simulink model "partialForceControlSim"  (Simulink 7.7)
settings: Solver=FixedStepDiscrete  StartTime=0.0  StopTime=inf  FixedStep=1  RelTol=1e-3
InitFcn:
  | initPartialForceControlSim;
values from neighbouring files (symbols this model uses):
  k_f = diag([k_f_linear k_f_rotatio])    [initPartialForceControl.m]
  k_pst = [ diag([k_pst_torso k_pst_arm k_pst_arm k_pst_leg k_pst_leg])    0*eye(25)   0*eye(25)]    [initPartialForceControl.m]    (also in initSharedMem.m)
  nc = 6    [initPartialForceControl.m]    (also in initSharedMem.m = 12)
  nj = 25    [initMonitor.m]    (also in initPartialForceControl.m; initSharedMem.m)
  Rf = [R, zeros(3,3); zeros(3,3), R]    [initMonitor.m]    (also in initPartialForceControl.m; initSharedMem.m)
undefined symbols (not defined in the file or in its folder): DiscIntNeverNeededParam
libraries: WBCLibrary x19, simulink x2, dspsigops x2
settings Model: Creator=daniele  LastModifiedBy=iron
settings DataIOCC: SignalLoggingSaveFormat=Dataset
settings DebuggingCC: FcnCallInpInsideContextMsg=Enable All

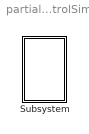
== system partialForceControlSim ==
  Subsystem : Subsystem  mask{robotName='icubGazeboSim', Ts=0.01, localName='dynamicBalancing'}
      mask prompts: robotName "robot name"; localName "module name"

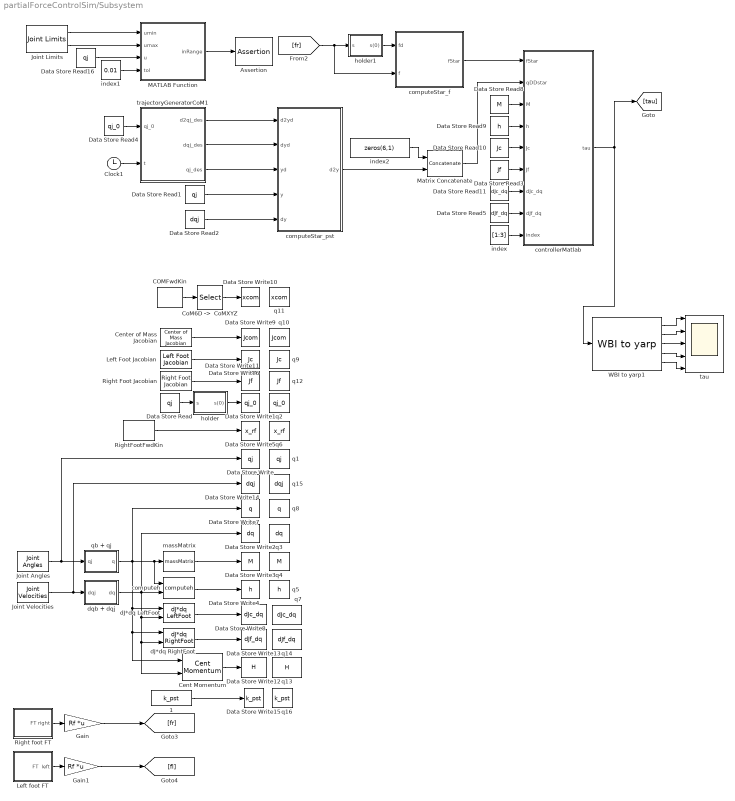
== system partialForceControlSim/Subsystem ==
  "    1" : Constant  Value=k_pst
  Assertion : Assertion  Enabled=on
  "COMFwdKin " : WBCLibrary/wholeBodyModel/Forward Kinematics/COMFwdKin   SystemSampleTime=-1  robotName=robotName  localName=localName
  Cent Momentum : WBCLibrary/wholeBodyModel/Dynamics/Cent Momentum  SystemSampleTime=-1  robotName=robotName  localName=localName
  Center of Mass Jacobian : WBCLibrary/wholeBodyModel/Jacobians/Center of Mass Jacobian  SystemSampleTime=-1  robotName=robotName  localName=localName
  Clock1 : Clock
  "CoM6D ->  CoMXYZ" : Selector  InputPortWidth=7  IndexOptions=Index vector (dialog)  Indices=[1 2 3]  OutputSizes=1
  Data Store Read : DataStoreRead  DataStoreName=qj
  Data Store Read1 : DataStoreRead  DataStoreName=qj
  Data Store Read10 : DataStoreRead  DataStoreName=Jc
  Data Store Read11 : DataStoreRead  DataStoreName=dJc_dq
  Data Store Read16 : DataStoreRead  DataStoreName=qj
  Data Store Read2 : DataStoreRead  DataStoreName=dqj
  Data Store Read3 : DataStoreRead  DataStoreName=Jf
  Data Store Read4 : DataStoreRead  DataStoreName=qj_0
  Data Store Read5 : DataStoreRead  DataStoreName=dJf_dq
  Data Store Read8 : DataStoreRead  DataStoreName=M
  Data Store Read9 : DataStoreRead  DataStoreName=h
  Data Store Write : DataStoreWrite  Priority=-1  DataStoreName=qj
  Data Store Write1 : DataStoreWrite  Priority=-1  DataStoreName=qj_0
  Data Store Write10 : DataStoreWrite  Priority=-1  DataStoreName=xcom
  Data Store Write11 : DataStoreWrite  Priority=-1  DataStoreName=Jf
  Data Store Write12 : DataStoreWrite  Priority=-1  DataStoreName=H
  Data Store Write13 : DataStoreWrite  Priority=-1  DataStoreName=dJf_dq
  Data Store Write14 : DataStoreWrite  Priority=-1  DataStoreName=dqj
  Data Store Write15 : DataStoreWrite  Priority=-1  DataStoreName=k_pst
  Data Store Write2 : DataStoreWrite  Priority=-1  DataStoreName=dq
  Data Store Write3 : DataStoreWrite  Priority=-1  DataStoreName=M
  Data Store Write4 : DataStoreWrite  Priority=-1  DataStoreName=h
  Data Store Write5 : DataStoreWrite  Priority=-1  DataStoreName=x_rf
  Data Store Write6 : DataStoreWrite  Priority=-1  DataStoreName=Jc
  Data Store Write7 : DataStoreWrite  Priority=-1  DataStoreName=q
  Data Store Write8 : DataStoreWrite  Priority=-1  DataStoreName=dJc_dq
  Data Store Write9 : DataStoreWrite  Priority=-1  DataStoreName=Jcom
  Gain : Gain  Gain=Rf  Multiplication=Matrix(K*u)
  Gain1 : Gain  Gain=Rf  Multiplication=Matrix(K*u)
  Joint Angles : WBCLibrary/wholeBodyStates/Joint Angles  SystemSampleTime=-1  robotName=robotName  localName=localName
  Joint Limits : WBCLibrary/wholeBodyModel/Joint Limits  SystemSampleTime=-1  robotName=robotName  localName=localName
  Joint Velocities : WBCLibrary/wholeBodyStates/Joint Velocities  SystemSampleTime=-1  robotName=robotName  localName=localName
  Left Foot Jacobian : WBCLibrary/wholeBodyModel/Jacobians/Left Foot Jacobian  SystemSampleTime=-1  robotName=robotName  localName=localName
  Left foot FT : Subsystem
  MATLAB Function : Stateflow chart  TreatAsAtomicUnit=on
  Matrix Concatenate : Concatenate  Mode=Multidimensional array
  Right Foot Jacobian : WBCLibrary/wholeBodyModel/Jacobians/Right Foot Jacobian  SystemSampleTime=-1  robotName=robotName  localName=localName
  Right foot FT : Subsystem
  RightFootFwdKin : WBCLibrary/wholeBodyModel/Forward Kinematics/RightFootFwdKin  SystemSampleTime=-1  robotName=robotName  localName=localName
  WBI to yarp1 : WBCLibrary/Utilities/WBI to yarp  SystemSampleTime=-1
  computeStar_f : Subsystem  mask{Kp=0, Kd=0, Ki=k_f(1:6,1:6)}
  computeStar_pst : Subsystem  mask{Kp=k_pst(1:25,1:25), Kd=k_pst(1:25,26:50), Ki=k_pst(1:25,51:75)}
  computeh : WBCLibrary/wholeBodyModel/Dynamics/computeh  SystemSampleTime=-1  val=7  robotname=robotName  localname=localName
  controllerMatlab : Stateflow chart  TreatAsAtomicUnit=on
  dJ*dq LeftFoot : WBCLibrary/wholeBodyModel/Dynamics/dJ*dq LeftFoot  SystemSampleTime=-1  val=9  robotName=robotName  localName=localName
  dJ*dq RightFoot : WBCLibrary/wholeBodyModel/Dynamics/dJ*dq RightFoot  SystemSampleTime=-1  val=9  robotName=robotName  localName=localName
  dqb + dqj : Subsystem
  holder : Subsystem
  holder1 : Subsystem
  index : Constant  Value=[1:3]  VectorParams1D=off
  index1 : Constant  Value=0.01  VectorParams1D=off
  index2 : Constant  Value=zeros(6,1)  VectorParams1D=off
  massMatrix : WBCLibrary/wholeBodyModel/Dynamics/massMatrix  SystemSampleTime=-1  val=8  robotname=robotName  localname=localName
  q1 : DataStoreMemory  Priority=-1  DataStoreName=qj  ReadBeforeWriteMsg=warning  WriteAfterWriteMsg=warning  WriteAfterReadMsg=warning  InitialValue=zeros(nj,1)  VectorParams1D=off  OutDataTypeStr=double
  q10 : DataStoreMemory  Priority=-1  DataStoreName=Jcom  ReadBeforeWriteMsg=warning  WriteAfterWriteMsg=warning  WriteAfterReadMsg=warning  InitialValue=zeros(6,nj+6)  VectorParams1D=off  OutDataTypeStr=double
  q11 : DataStoreMemory  Priority=-1  DataStoreName=xcom  ReadBeforeWriteMsg=warning  WriteAfterWriteMsg=warning  WriteAfterReadMsg=warning  InitialValue=zeros(3,1)  VectorParams1D=off  OutDataTypeStr=double
  q12 : DataStoreMemory  Priority=-1  DataStoreName=Jf  ReadBeforeWriteMsg=warning  WriteAfterWriteMsg=warning  WriteAfterReadMsg=warning  InitialValue=zeros(nc,nj+6)  VectorParams1D=off  OutDataTypeStr=double
  q13 : DataStoreMemory  Priority=-1  DataStoreName=H  ReadBeforeWriteMsg=warning  WriteAfterWriteMsg=warning  WriteAfterReadMsg=warning  InitialValue=zeros(6,1)  VectorParams1D=off  OutDataTypeStr=double
  q14 : DataStoreMemory  Priority=-1  DataStoreName=dJf_dq  ReadBeforeWriteMsg=warning  WriteAfterWriteMsg=warning  WriteAfterReadMsg=warning  InitialValue=zeros(nc,1)  VectorParams1D=off  OutDataTypeStr=double
  q15 : DataStoreMemory  Priority=-1  DataStoreName=dqj  ReadBeforeWriteMsg=warning  WriteAfterWriteMsg=warning  WriteAfterReadMsg=warning  InitialValue=zeros(nj,1)  VectorParams1D=off  OutDataTypeStr=double
  q16 : DataStoreMemory  Priority=-1  DataStoreName=k_pst  ReadBeforeWriteMsg=warning  WriteAfterWriteMsg=warning  WriteAfterReadMsg=warning  InitialValue=k_pst  VectorParams1D=off  OutDataTypeStr=double
  q2 : DataStoreMemory  Priority=-1  DataStoreName=qj_0  ReadBeforeWriteMsg=warning  WriteAfterWriteMsg=warning  WriteAfterReadMsg=warning  InitialValue=zeros(nj,1)  VectorParams1D=off  OutDataTypeStr=double
  q3 : DataStoreMemory  Priority=-1  DataStoreName=dq  ReadBeforeWriteMsg=warning  WriteAfterWriteMsg=warning  WriteAfterReadMsg=warning  InitialValue=zeros(nj+6,1)  VectorParams1D=off  OutDataTypeStr=double
  q4 : DataStoreMemory  Priority=-1  DataStoreName=M  ReadBeforeWriteMsg=warning  WriteAfterWriteMsg=warning  WriteAfterReadMsg=warning  InitialValue=zeros(nj+6,nj+6)  VectorParams1D=off  OutDataTypeStr=double
  q5 : DataStoreMemory  Priority=-1  DataStoreName=h  ReadBeforeWriteMsg=warning  WriteAfterWriteMsg=warning  WriteAfterReadMsg=warning  InitialValue=zeros(nj+6,1)  VectorParams1D=off  OutDataTypeStr=double
  q6 : DataStoreMemory  Priority=-1  DataStoreName=x_rf  ReadBeforeWriteMsg=warning  WriteAfterWriteMsg=warning  WriteAfterReadMsg=warning  InitialValue=zeros(7,1)  VectorParams1D=off  OutDataTypeStr=double
  q7 : DataStoreMemory  Priority=-1  DataStoreName=dJc_dq  ReadBeforeWriteMsg=warning  WriteAfterWriteMsg=warning  WriteAfterReadMsg=warning  InitialValue=zeros(nc,1)  VectorParams1D=off  OutDataTypeStr=double
  q8 : DataStoreMemory  Priority=-1  DataStoreName=q  ReadBeforeWriteMsg=warning  WriteAfterWriteMsg=warning  WriteAfterReadMsg=warning  InitialValue=zeros(nj+16,1)  VectorParams1D=off  OutDataTypeStr=double
  q9 : DataStoreMemory  Priority=-1  DataStoreName=Jc  ReadBeforeWriteMsg=warning  WriteAfterWriteMsg=warning  WriteAfterReadMsg=warning  InitialValue=zeros(nc,nj+6)  VectorParams1D=off  OutDataTypeStr=double
  qb + qj : Subsystem
  tau : Scope  NumInputPorts=5
      settings: TimeRange=2000  YMin=-8~-1.75~-1.75~-2~-2  YMax=1~1.25~1.25~6~6
  trajectoryGeneratorCoM1 : Stateflow chart  TreatAsAtomicUnit=on
  wires:
  Clock1/1 -> trajectoryGeneratorCoM1/2(t)
  Data Store Read4/1 -> trajectoryGeneratorCoM1/1(qj_0)
  trajectoryGeneratorCoM1/1(d2qj_des) -> computeStar_pst/1(d2yd)
  trajectoryGeneratorCoM1/2(dqj_des) -> computeStar_pst/2(dyd)
  trajectoryGeneratorCoM1/3(qj_des) -> computeStar_pst/3(yd)
  Data Store Read1/1 -> computeStar_pst/4(y)
  Data Store Read2/1 -> computeStar_pst/5(dy)
  Joint Limits/1 -> MATLAB Function/1(umin)
  Joint Limits/2 -> MATLAB Function/2(umax)
  Data Store Read16/1 -> MATLAB Function/3(u)
  index1/1 -> MATLAB Function/4(tol)
  MATLAB Function/1(inRange) -> Assertion/1
  index2/1 -> Matrix Concatenate/1
  computeStar_pst/1(d2y) -> Matrix Concatenate/2
  Matrix Concatenate/1 -> controllerMatlab/2(qDDstar)
  index/1 -> controllerMatlab/9(index)
  controllerMatlab/1(tau) -> WBI to yarp1/1, [tau]
  Data Store Read8/1 -> controllerMatlab/3(M)
  Data Store Read9/1 -> controllerMatlab/4(h)
  Data Store Read10/1 -> controllerMatlab/5(Jc)
  Data Store Read11/1 -> controllerMatlab/7(dJc_dq)
  [fr] -> holder1/1(s), computeStar_f/2(f)
  holder1/1(s(0)) -> computeStar_f/1(fd)
  computeStar_f/1(fStar) -> controllerMatlab/1(fStar)
  Data Store Read3/1 -> controllerMatlab/6(Jf)
  Data Store Read5/1 -> controllerMatlab/8(dJf_dq)
  qb + qj/1(q) -> massMatrix/1, computeh/1, Data Store Write7/1, dJ*dq LeftFoot/1, Cent Momentum/1, dJ*dq RightFoot/1
  dqb + dqj/1(dq) -> computeh/2, Data Store Write2/1, dJ*dq LeftFoot/2, Cent Momentum/2, dJ*dq RightFoot/2
  Data Store Read/1 -> holder/1(s)
  holder/1(s(0)) -> Data Store Write1/1
  massMatrix/1 -> Data Store Write3/1
  computeh/1 -> Data Store Write4/1
  Joint Velocities/1 -> dqb + dqj/1(dqj), Data Store Write14/1
  RightFootFwdKin/1 -> Data Store Write5/1
  Center of Mass Jacobian/1 -> Data Store Write9/1
  "COMFwdKin "/1 -> "CoM6D ->  CoMXYZ"/1
  "CoM6D ->  CoMXYZ"/1 -> Data Store Write10/1
  Cent Momentum/1 -> Data Store Write12/1
  Joint Angles/1 -> qb + qj/1(qj), Data Store Write/1
  "    1"/1 -> Data Store Write15/1
  Left Foot Jacobian/1 -> Data Store Write6/1
  Right Foot Jacobian/1 -> Data Store Write11/1
  dJ*dq LeftFoot/1 -> Data Store Write8/1
  dJ*dq RightFoot/1 -> Data Store Write13/1
  Right foot FT/1(FT right) -> Gain/1
  Left foot FT/1(FT  left) -> Gain1/1
  Gain/1 -> [fr]
  Gain1/1 -> [fl]
  WBI to yarp1/1 -> tau/1
  WBI to yarp1/2 -> tau/2
  WBI to yarp1/3 -> tau/3
  WBI to yarp1/4 -> tau/4
  WBI to yarp1/5 -> tau/5

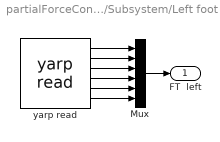
== system partialForceControlSim/Subsystem/Left foot FT ==
  Mux : Mux  Inputs=6
  yarp read : WBCLibrary/Utilities/yarp read  from=['/' robotName '/left_foot/analog:o']  to='...'  num=6
  FT  left : Outport
  wires:
  yarp read/1 -> Mux/1
  yarp read/2 -> Mux/2
  yarp read/3 -> Mux/3
  yarp read/4 -> Mux/4
  yarp read/5 -> Mux/5
  yarp read/6 -> Mux/6
  Mux/1 -> FT  left/1

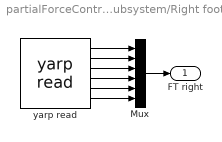
== system partialForceControlSim/Subsystem/Right foot FT ==
  Mux : Mux  Inputs=6
  yarp read : WBCLibrary/Utilities/yarp read  from=['/' robotName '/right_foot/analog:o']  to='...'  num=6
  FT right : Outport
  wires:
  yarp read/1 -> Mux/1
  yarp read/2 -> Mux/2
  yarp read/3 -> Mux/3
  yarp read/4 -> Mux/4
  yarp read/5 -> Mux/5
  yarp read/6 -> Mux/6
  Mux/1 -> FT right/1

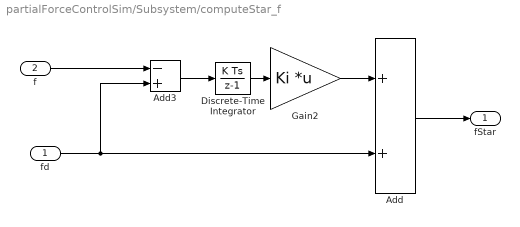
== system partialForceControlSim/Subsystem/computeStar_f ==
  fd : Inport
  f : Inport  Port=2
  Add : Sum
  Add3 : Sum  Inputs=-+
  Discrete-Time Integrator : DiscreteIntegrator  ICPrevOutput=DiscIntNeverNeededParam  ICPrevScaledInput=DiscIntNeverNeededParam
  Gain2 : Gain  Gain=Ki  Multiplication=Matrix(K*u)
  fStar : Outport
  wires:
  Add/1 -> fStar/1
  f/1 -> Add3/1
  Add3/1 -> Discrete-Time Integrator/1
  Discrete-Time Integrator/1 -> Gain2/1
  Gain2/1 -> Add/1
  fd/1 -> Add3/2, Add/2

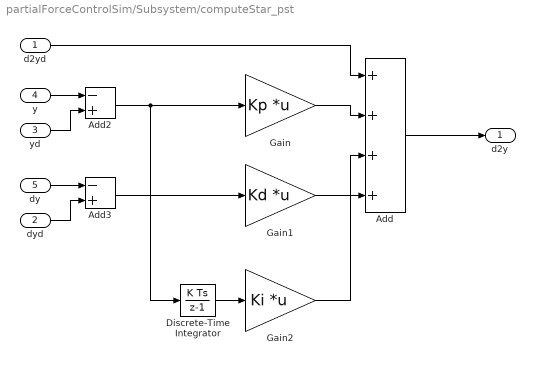
== system partialForceControlSim/Subsystem/computeStar_pst ==
  d2yd : Inport
  dyd : Inport  Port=2
  yd : Inport  Port=3
  y : Inport  Port=4
  dy : Inport  Port=5
  Add : Sum  Inputs=++++
  Add2 : Sum  Inputs=-+
  Add3 : Sum  Inputs=-+
  Discrete-Time Integrator : DiscreteIntegrator  ICPrevOutput=DiscIntNeverNeededParam  ICPrevScaledInput=DiscIntNeverNeededParam
  Gain : Gain  Gain=Kp  Multiplication=Matrix(K*u)
  Gain1 : Gain  Gain=Kd  Multiplication=Matrix(K*u)
  Gain2 : Gain  Gain=Ki  Multiplication=Matrix(K*u)
  d2y : Outport
  wires:
  Discrete-Time Integrator/1 -> Gain2/1
  dyd/1 -> Add3/2
  yd/1 -> Add2/2
  d2yd/1 -> Add/1
  Add3/1 -> Gain1/1
  dy/1 -> Add3/1
  Add2/1 -> Discrete-Time Integrator/1, Gain/1
  y/1 -> Add2/1
  Add/1 -> d2y/1
  Gain2/1 -> Add/4
  Gain1/1 -> Add/3
  Gain/1 -> Add/2

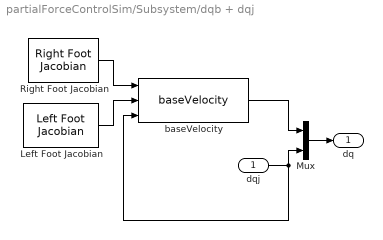
== system partialForceControlSim/Subsystem/dqb + dqj ==
  dqj : Inport
  Left Foot Jacobian : WBCLibrary/wholeBodyModel/Jacobians/Left Foot Jacobian  SystemSampleTime=-1  robotName=robotName  localName=localName
  Mux : Mux  Inputs=2
  Right Foot Jacobian : WBCLibrary/wholeBodyModel/Jacobians/Right Foot Jacobian  SystemSampleTime=-1  robotName=robotName  localName=localName
  baseVelocity : WBCLibrary/Utilities/baseVelocity  SystemSampleTime=-1
  dq : Outport
  wires:
  Left Foot Jacobian/1 -> baseVelocity/2
  Right Foot Jacobian/1 -> baseVelocity/1
  baseVelocity/1 -> Mux/1
  dqj/1 -> baseVelocity/3, Mux/2
  Mux/1 -> dq/1

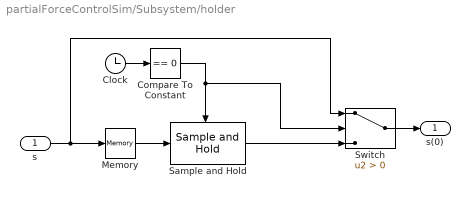
== system partialForceControlSim/Subsystem/holder ==
  s : Inport
  Clock : Clock
      settings: Decimation=10
  Compare To Constant : simulink/Logic and Bit Operations/Compare To Constant  SystemSampleTime=-1  relop===  const=0  LogicOutDataTypeMode=boolean
  Memory : Memory
  Sample and Hold : dspsigops/Sample and Hold  SystemSampleTime=-1  trig=Falling edge  initCond=0  latchinput=off
  Switch : Switch  Criteria=u2 > Threshold
  s(0) : Outport
  wires:
  s/1 -> Switch/1, Memory/1
  Clock/1 -> Compare To Constant/1
  Compare To Constant/1 -> Sample and Hold/Trigger, Switch/2
  Sample and Hold/1 -> Switch/3
  Switch/1 -> s(0)/1
  Memory/1 -> Sample and Hold/1

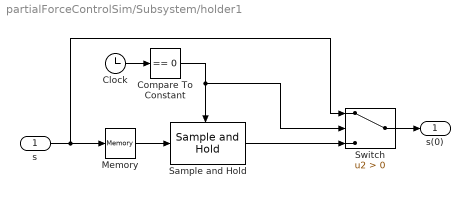
== system partialForceControlSim/Subsystem/holder1 ==
  s : Inport
  Clock : Clock
      settings: Decimation=10
  Compare To Constant : simulink/Logic and Bit Operations/Compare To Constant  SystemSampleTime=-1  relop===  const=0  LogicOutDataTypeMode=boolean
  Memory : Memory
  Sample and Hold : dspsigops/Sample and Hold  SystemSampleTime=-1  trig=Falling edge  initCond=0  latchinput=off
  Switch : Switch  Criteria=u2 > Threshold
  s(0) : Outport
  wires:
  Memory/1 -> Sample and Hold/1
  Switch/1 -> s(0)/1
  Sample and Hold/1 -> Switch/3
  Compare To Constant/1 -> Switch/2, Sample and Hold/Trigger
  Clock/1 -> Compare To Constant/1
  s/1 -> Memory/1, Switch/1

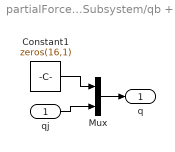
== system partialForceControlSim/Subsystem/qb + qj ==
  qj : Inport
  Constant1 : Constant  Value=zeros(16,1)
  Mux : Mux  Inputs=2
  q : Outport
  wires:
  Mux/1 -> q/1
  Constant1/1 -> Mux/1
  qj/1 -> Mux/2

== matlab function Subsystem/controllerMatlab ==
  data: fStar input double; qDDstar input double; M input double; h input double; Jc input double; Jf input double; tau output double; dJc_dq input double; dJf_dq input double; index input double
function tau  = computeTau(fStar, qDDstar, M, h, Jc, Jf, dJc_dq, dJf_dq, index)
%#codegen

PINV_TOL = 1e-5;

[~,~,V] = svd(Jc);
V2      = V(:, 7:end);
Jcf     = [Jc; Jf];
dJcf_dq = [dJc_dq; dJf_dq];

[mc, nc] = size(Jcf);
n        = nc - 6;

S        = [zeros(n,6), eye(n)];

% Definition of reference accelerations for CoM and Joints that ensure
% stabilization of desired trajectories xDcomDes and qDes 

J0     = [zeros(n,6), eye(n)];
J1     = J0(index,:);
J2     = Jcf;

dJ1_dq = zeros(length(index), 1);
dJ2_dq = dJcf_dq;

d2x2   = zeros(mc,1);
d2x1   = qDDstar(6+index);

 Np3   = eye(n+6,n+6);
d2q3   = zeros(n+6,1);
d2q0   = qDDstar;
% q_star =   -5.*ones(size(q_star));

% We apply the recursion in Del Prete Ph.D. thesis (6.27)
% with N = 2 and with a redefinition Npi -> Npi+1.
%
% i = 2 = N
% d2q_2 = pinv(Jcf)*(-dJcf_dq);
% N_p2  = I
%
% i = 1
% d2q_1 = d2q_2 + JiSBarN_p1Pinv*(d2x_i - Ji SBar d2q_2)
% N_p1  = N_p2 - pinv(JcSbarN_p2)*JcSbarN_p2
%
% d2q_s = d2q_1 + N_p0*d2q_0
% N_p0  = N_p1 - pinv(Ji*Sbar*N_p1)*Ji*Sbar*N_p1


d2q2 = d2q3 + pinv(J2* Np3, PINV_TOL) * (d2x2 - dJ2_dq - J2*d2q3);
Np2  = Np3 - pinv(J2* Np3, PINV_TOL)*J2*Np3;

d2q1 = d2q2 + pinv(J1* Np2, PINV_TOL) * (d2x1 - dJ1_dq - J1*d2q2);
Np1  = Np2 - pinv(J1* Np2, PINV_TOL)*J1*Np2;

d2q_s = d2q1 + Np1 * d2q0;
tau   = pinv(V2'*S', PINV_TOL) * V2' * (M*d2q_s + h - Jf'*fStar);

== matlab function Subsystem/MATLAB Function ==
  data: umin input double; umax input double; u input double; inRange output double; tol input double
function inRange = checkRange(umin, umax, u, tol)
%#codegen

res = u < umin + tol | u > umax - tol;
res = sum(res);
if res==0
    inRange = 1;
else
    inRange = 0;
    u < umin + tol | u > umax - tol
end

== matlab function Subsystem/trajectoryGeneratorCoM1 ==
  data: d2qj_des output double; dqj_des output double; qj_des output double; qj_0 input double; t input double; Jcom data_store_memory double; dq data_store_memory double
function [d2qj_des, dqj_des, qj_des]  = trajGen(qj_0,t)
%#codegen


qj_des    = qj_0;
qj_des(25)= qj_des(25)+0.1*sin(t*0.003);
% qj_des(17)= qj_des(17)+0.15*sin(t*0.001);
% qj_des(23)= qj_des(23)+0.15*sin(t*0.001);
dqj_des   = zeros(size(qj_0));
d2qj_des  = zeros(size(qj_0));
